simulink model "s0312b"  (Simulink 6.0)
settings: Solver=ode3  SolverMode=SingleTasking  StartTime=0.0  StopTime=900  FixedStep=1  MaxStep=1  RelTol=1e-3  AbsTol=1e-6
values from neighbouring files (symbols this model uses):
  T1 = 3*T1    (= 0.3)    [m0203.m]    (also in m0204.m = 0.1; m0205.m = 0.1; m0207.m = 0.1; m0221d.m = 1/a0)
  ydach = 1    [m0305.m]    (also in m0306.m; m0311.m; m0312b.m; m0313.m)
settings Model: LastModifiedBy=Froriep
settings DataIOCC: LimitDataPoints=off  SaveOutput=off  SaveTime=off
settings OptimizationCC: BooleanDataType=off
settings DebuggingCC: SolverPrmCheckMsg=none
settings HardwareCC: TargetUnknown=on
settings GRTTargetCC: ModelReferenceCompliant=off  MatFileLogging=off

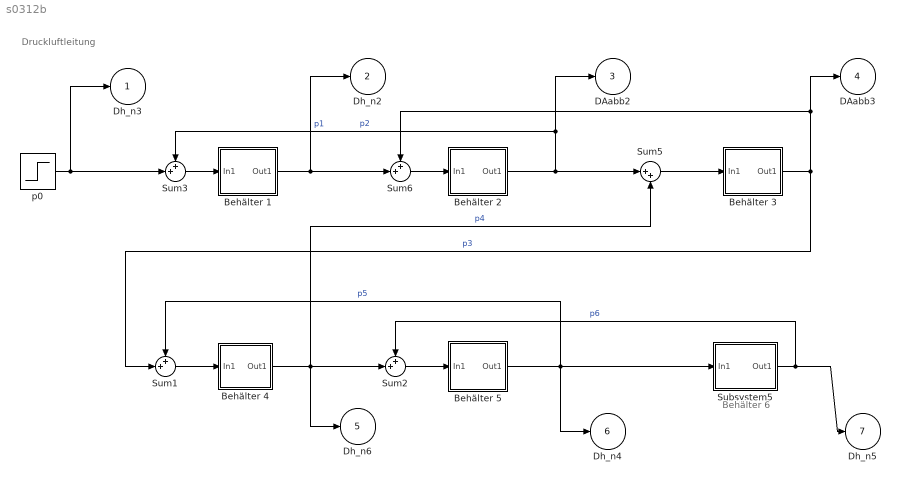
== system s0312b ==
  note: Behälter 6
  note: Druckluftleitung
  Behälter 1 : Subsystem
  Behälter 2 : Subsystem
  Behälter 3 : Subsystem
  Behälter 4 : Subsystem
  Behälter 5 : Subsystem
  Subsystem5 : Subsystem
  Sum{1..3,6} (4 alike) : Sum  Inputs=++|
  Sum5 : Sum  Inputs=|++
  p0 : Step  Time=0  After=ydach  SampleTime=0
  Dh_n3 : Outport
  Dh_n2 : Outport  Port=2
  DAabb2 : Outport  Port=3
  DAabb3 : Outport  Port=4
  Dh_n6 : Outport  Port=5
  Dh_n4 : Outport  Port=6
  Dh_n5 : Outport  Port=7
  wires:
  Behälter 1/1(Out1) -> Dh_n2/1, Sum6/2  "p1"
  Sum3/1 -> Behälter 1/1(In1)
  p0/1 -> Dh_n3/1, Sum3/2
  Behälter 3/1(Out1) -> Sum6/1, DAabb3/1, Sum1/2  "p3"
  Sum6/1 -> Behälter 2/1(In1)
  Behälter 2/1(Out1) -> Sum3/1, DAabb2/1, Sum5/1  "p2"
  Sum5/1 -> Behälter 3/1(In1)
  Behälter 4/1(Out1) -> Sum5/2, Dh_n6/1, Sum2/2  "p4"
  Sum1/1 -> Behälter 4/1(In1)
  Behälter 5/1(Out1) -> Dh_n4/1, Subsystem5/1(In1), Sum1/1  "p5"
  Sum2/1 -> Behälter 5/1(In1)
  Subsystem5/1(Out1) -> Dh_n5/1, Sum2/1  "p6"

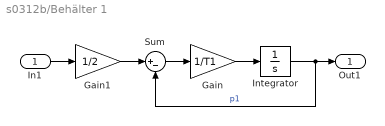
== system s0312b/Behälter 1 ==
  In1 : Inport  Port=1  LatchInput=off
  Gain : Gain  Gain=1/T1
  Gain1 : Gain  Gain=1/2
  Integrator : Integrator
  Sum : Sum  Inputs=|+-
  Out1 : Outport
  wires:
  In1/1 -> Gain1/1
  Gain/1 -> Integrator/1
  Sum/1 -> Gain/1
  Integrator/1 -> Out1/1, Sum/2  "p1"
  Gain1/1 -> Sum/1

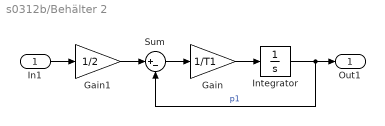
== system s0312b/Behälter 2 ==
  In1 : Inport  Port=1  LatchInput=off
  Gain : Gain  Gain=1/T1
  Gain1 : Gain  Gain=1/2
  Integrator : Integrator
  Sum : Sum  Inputs=|+-
  Out1 : Outport
  wires:
  Gain1/1 -> Sum/1
  Integrator/1 -> Sum/2, Out1/1  "p1"
  Sum/1 -> Gain/1
  Gain/1 -> Integrator/1
  In1/1 -> Gain1/1

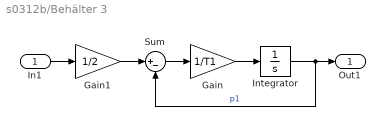
== system s0312b/Behälter 3 ==
  In1 : Inport  Port=1  LatchInput=off
  Gain : Gain  Gain=1/T1
  Gain1 : Gain  Gain=1/2
  Integrator : Integrator
  Sum : Sum  Inputs=|+-
  Out1 : Outport
  wires:
  In1/1 -> Gain1/1
  Gain/1 -> Integrator/1
  Sum/1 -> Gain/1
  Integrator/1 -> Out1/1, Sum/2  "p1"
  Gain1/1 -> Sum/1

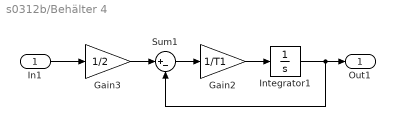
== system s0312b/Behälter 4 ==
  In1 : Inport  Port=1  LatchInput=off
  Gain2 : Gain  Gain=1/T1
  Gain3 : Gain  Gain=1/2
  Integrator1 : Integrator
  Sum1 : Sum  Inputs=|+-
  Out1 : Outport
  wires:
  Gain2/1 -> Integrator1/1
  Sum1/1 -> Gain2/1
  Integrator1/1 -> Sum1/2, Out1/1
  Gain3/1 -> Sum1/1
  In1/1 -> Gain3/1

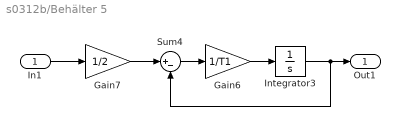
== system s0312b/Behälter 5 ==
  In1 : Inport  Port=1  LatchInput=off
  Gain6 : Gain  Gain=1/T1
  Gain7 : Gain  Gain=1/2
  Integrator3 : Integrator
  Sum4 : Sum  Inputs=|+-
  Out1 : Outport
  wires:
  Gain6/1 -> Integrator3/1
  Sum4/1 -> Gain6/1
  Integrator3/1 -> Sum4/2, Out1/1
  Gain7/1 -> Sum4/1
  In1/1 -> Gain7/1

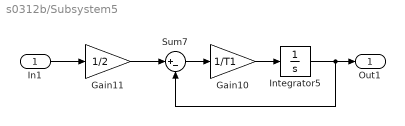
== system s0312b/Subsystem5 ==
  In1 : Inport  Port=1  LatchInput=off
  Gain10 : Gain  Gain=1/T1
  Gain11 : Gain  Gain=1/2
  Integrator5 : Integrator
  Sum7 : Sum  Inputs=|+-
  Out1 : Outport
  wires:
  Gain10/1 -> Integrator5/1
  Sum7/1 -> Gain10/1
  Integrator5/1 -> Sum7/2, Out1/1
  Gain11/1 -> Sum7/1
  In1/1 -> Gain11/1
